simulink model "control_PD"  (R2015a)
settings: Solver=ode4  StartTime=0.0  StopTime=10.0  FixedStep=1e-3  RelTol=1e-3
settings Model: Creator=Sala6  LastModifiedBy=Jesus

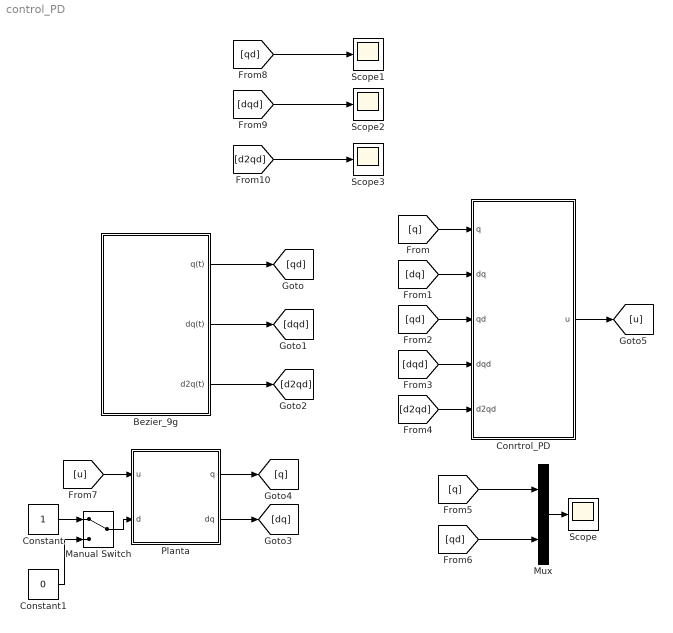
== system control_PD ==
  Bezier_9g : Subsystem  mask{t0=4.5, t1=5.5, q0=4, q1=8}
      mask prompts: t0 "Tiempo de transición"; t1 "Tiempo de transición"; q0 "Posición inicial"; q1 "Posición final"
      mask init:
      | gamma0=126;
      | gamma1=420;
      | gamma2=540;
      | gamma3=315;
      | gamma4=70;
  Conrtrol_PD : Subsystem  mask{J=.02, B=.6, z=5, wn=40}
      mask prompts: J "Inercia efectiva"; B "Amortiguamiento"; z "Amortiguamiento deseado"; wn "Frecuencia natural deseada"
      mask init:
      | kd=2*z*wn-(B/J);
      | kp=wn^2;
  Constant : Constant
  Constant1 : Constant  Value=0
  Manual Switch : ManualSwitch
  Mux : Mux  Inputs=2
  Planta : Subsystem  mask{J=.02, B=.6, q0=pi/3, dq0=-pi}
      mask prompts: J "Inercia efectiva"; B "Amortiguamiento"; q0 "Posicion inicial"; dq0 "Velocidad inicial"
  Scope{,1..3} (4 alike) : Scope
      Scope2 settings: SaveName=ScopeData2
      Scope3 settings: SaveName=ScopeData3
  wires:
  Bezier_9g/1(q(t)) -> [qd]
  Bezier_9g/2("dq(t) ") -> [dqd]
  Bezier_9g/3(d2q(t)) -> [d2qd]
  Planta/2(dq) -> [dq]
  Planta/1(q) -> [q]
  [q] -> Conrtrol_PD/1(q)
  [dq] -> Conrtrol_PD/2(dq)
  [qd] -> Conrtrol_PD/3(qd)
  [dqd] -> Conrtrol_PD/4(dqd)
  [d2qd] -> Conrtrol_PD/5(d2qd)
  Conrtrol_PD/1(u) -> [u]
  Mux/1 -> Scope/1
  [q] -> Mux/1
  [qd] -> Mux/2
  Constant/1 -> Manual Switch/1
  Constant1/1 -> Manual Switch/2
  [qd] -> Scope1/1
  [dqd] -> Scope2/1
  [d2qd] -> Scope3/1
  [u] -> Planta/1(u)
  Manual Switch/1 -> Planta/2(d)

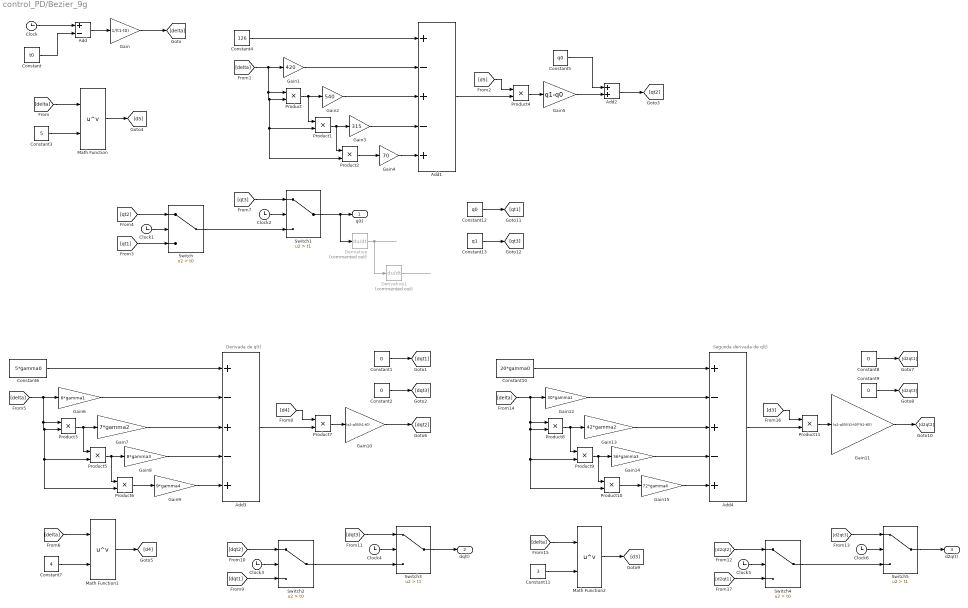
== system control_PD/Bezier_9g ==
  note: Segunda derivada de q(t)
  note: Derivada de q(t)
  Add : Sum  Inputs=+-
  Add1 : Sum  Inputs=+-+-+
  Add2 : Sum
  Add3 : Sum  Inputs=+-+-+
  Add4 : Sum  Inputs=+-+-+
  Clock{,1..6} (7 alike) : Clock
  Constant : Constant  Value=t0
  Constant{1..2,8..9} (4 alike) : Constant  Value=0
  Constant10 : Constant  Value=20*gamma0
  Constant11 : Constant  Value=3
  Constant12 : Constant  Value=q0
  Constant13 : Constant  Value=q1
  Constant3 : Constant  Value=5
  Constant4 : Constant  Value=126
  Constant5 : Constant  Value=q0
  Constant6 : Constant  Value=5*gamma0
  Constant7 : Constant  Value=4
  Derivative : Derivative  Commented=on
  Derivative1 : Derivative  Commented=on
  Gain : Gain  Gain=1/(t1-t0)
  Gain1 : Gain  Gain=420
  Gain10 : Gain  Gain=(q1-q0)/(t1-t0)
  Gain11 : Gain  Gain=(q1-q0)/((t1-t0)*(t1-t0))
  Gain12 : Gain  Gain=30*gamma1
  Gain13 : Gain  Gain=42*gamma2
  Gain14 : Gain  Gain=56*gamma3
  Gain15 : Gain  Gain=72*gamma4
  Gain2 : Gain  Gain=540
  Gain3 : Gain  Gain=315
  Gain4 : Gain  Gain=70
  Gain5 : Gain  Gain=q1-q0
  Gain6 : Gain  Gain=6*gamma1
  Gain7 : Gain  Gain=7*gamma2
  Gain8 : Gain  Gain=8*gamma3
  Gain9 : Gain  Gain=9*gamma4
  Math Function : Math  Operator=pow  SaturateOnIntegerOverflow=on
  Math Function1 : Math  Operator=pow  SaturateOnIntegerOverflow=on
  Math Function2 : Math  Operator=pow  SaturateOnIntegerOverflow=on
  Product{,1..11} (12 alike) : Product
  Switch : Switch  Criteria=u2 > Threshold  Threshold=t0
  Switch1 : Switch  Criteria=u2 > Threshold  Threshold=t1
  Switch2 : Switch  Criteria=u2 > Threshold  Threshold=t0
  Switch3 : Switch  Criteria=u2 > Threshold  Threshold=t1
  Switch4 : Switch  Criteria=u2 > Threshold  Threshold=t0
  Switch5 : Switch  Criteria=u2 > Threshold  Threshold=t1
  q(t) : Outport
  "dq(t) " : Outport  Port=2
  d2q(t) : Outport  Port=3
  wires:
  Constant12/1 -> [qt1]
  Constant13/1 -> [qt3]
  Switch5/1 -> d2q(t)/1
  Switch4/1 -> Switch5/3
  [d2qt2] -> Switch4/1
  [d2qt1] -> Switch4/3
  Clock6/1 -> Switch5/2
  [d2qt3] -> Switch5/1
  Clock5/1 -> Switch4/2
  Gain11/1 -> [d2qt2]
  Product11/1 -> Gain11/1
  [d3] -> Product11/1
  Add4/1 -> Product11/2
  Math Function2/1 -> [d3]
  Constant11/1 -> Math Function2/2
  [delta] -> Math Function2/1
  Gain13/1 -> Add4/3
  Gain15/1 -> Add4/5
  Gain14/1 -> Add4/4
  Constant10/1 -> Add4/1
  Gain12/1 -> Add4/2
  Product8/1 -> Gain13/1, Product9/1
  [delta] -> Gain12/1, Product8/1, Product8/2, Product9/2, Product10/2
  Product9/1 -> Gain14/1, Product10/1
  Product10/1 -> Gain15/1
  Constant8/1 -> [d2qt1]
  Constant9/1 -> [d2qt3]
  Switch3/1 -> "dq(t) "/1
  Switch2/1 -> Switch3/3
  [dqt2] -> Switch2/1
  [dqt1] -> Switch2/3
  Clock4/1 -> Switch3/2
  [dqt3] -> Switch3/1
  Clock3/1 -> Switch2/2
  Gain10/1 -> [dqt2]
  Product7/1 -> Gain10/1
  [d4] -> Product7/1
  Add3/1 -> Product7/2
  Math Function1/1 -> [d4]
  Constant7/1 -> Math Function1/2
  [delta] -> Math Function1/1
  Gain7/1 -> Add3/3
  Gain9/1 -> Add3/5
  Gain8/1 -> Add3/4
  Constant6/1 -> Add3/1
  Gain6/1 -> Add3/2
  Product3/1 -> Product5/1, Gain7/1
  [delta] -> Product6/2, Product5/2, Product3/2, Product3/1, Gain6/1
  Product5/1 -> Product6/1, Gain8/1
  Product6/1 -> Gain9/1
  Derivative1/1 -> ?
  Derivative/1 -> Derivative1/1
  Switch1/1 -> q(t)/1, Derivative/1
  Switch/1 -> Switch1/3
  Math Function/1 -> [d5]
  [qt2] -> Switch/1
  [qt1] -> Switch/3
  Gain5/1 -> Add2/2
  Clock2/1 -> Switch1/2
  [qt3] -> Switch1/1
  Clock1/1 -> Switch/2
  Product4/1 -> Gain5/1
  Constant5/1 -> Add2/1
  Add2/1 -> [qt2]
  [d5] -> Product4/1
  Gain2/1 -> Add1/3
  Gain4/1 -> Add1/5
  Gain3/1 -> Add1/4
  Constant4/1 -> Add1/1
  Gain1/1 -> Add1/2
  Product/1 -> Gain2/1, Product1/1
  [delta] -> Gain1/1, Product/1, Product/2, Product1/2, Product2/2
  Add1/1 -> Product4/2
  Product1/1 -> Gain3/1, Product2/1
  Product2/1 -> Gain4/1
  Constant3/1 -> Math Function/2
  Clock/1 -> Add/1
  [delta] -> Math Function/1
  Constant1/1 -> [dqt1]
  Constant2/1 -> [dqt3]
  Add/1 -> Gain/1
  Gain/1 -> [delta]
  Constant/1 -> Add/2

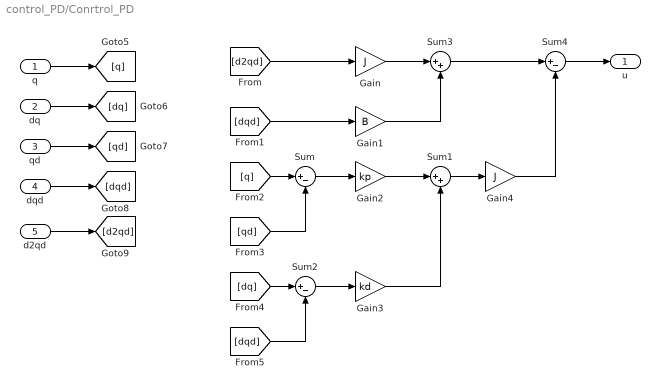
== system control_PD/Conrtrol_PD ==
  q : Inport
  dq : Inport  Port=2
  qd : Inport  Port=3
  dqd : Inport  Port=4
  d2qd : Inport  Port=5
  Gain : Gain  Gain=J
  Gain1 : Gain  Gain=B
  Gain2 : Gain  Gain=kp
  Gain3 : Gain  Gain=kd
  Gain4 : Gain  Gain=J
  Sum : Sum  Inputs=|+-
  Sum1 : Sum  Inputs=|++
  Sum2 : Sum  Inputs=|+-
  Sum3 : Sum  Inputs=|++
  Sum4 : Sum  Inputs=|+-
  u : Outport
  wires:
  dqd/1 -> [dqd]
  qd/1 -> [qd]
  dq/1 -> [dq]
  d2qd/1 -> [d2qd]
  q/1 -> [q]
  [dqd] -> Gain1/1
  [d2qd] -> Gain/1
  Sum/1 -> Gain2/1
  [q] -> Sum/1
  [qd] -> Sum/2
  Gain2/1 -> Sum1/1
  Sum2/1 -> Gain3/1
  [dq] -> Sum2/1
  [dqd] -> Sum2/2
  Gain3/1 -> Sum1/2
  Gain/1 -> Sum3/1
  Gain1/1 -> Sum3/2
  Sum1/1 -> Gain4/1
  Sum3/1 -> Sum4/1
  Gain4/1 -> Sum4/2
  Sum4/1 -> u/1

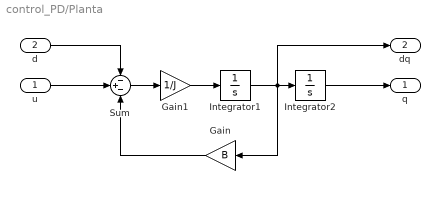
== system control_PD/Planta ==
  u : Inport
  d : Inport  Port=2
  Gain : Gain  Gain=B
  Gain1 : Gain  Gain=1/J
  Integrator1 : Integrator  InitialCondition=dq0
  Integrator2 : Integrator  InitialCondition=q0
  Sum : Sum  Inputs=-+-
  q : Outport
  dq : Outport  Port=2
  wires:
  Integrator1/1 -> dq/1, Gain/1, Integrator2/1
  Gain1/1 -> Integrator1/1
  Sum/1 -> Gain1/1
  d/1 -> Sum/1
  Gain/1 -> Sum/3
  u/1 -> Sum/2
  Integrator2/1 -> q/1
